simulink model "vco"  (R2019b)
settings: Solver=ode113  StartTime=0.0  StopTime=1e-6  RelTol=1e-3
values from neighbouring files (symbols this model uses):
  fs = fB*2    (= 10000000)    [vco_counter_m.m]    (also in vco_m.m = 1600000000)
  fvco = 1000e6    (= 1000000000)    [vco_counter_m.m]    (also in vco_m.m = 1600000000)
  ts = 1/fs    (= 1e-07)    [vco_counter_m.m]    (also in vco_m.m = 6.25e-10)
  tsys_res = 1e-11    [vco_counter_m.m]    (also in vco_m.m = 6.25e-10)
  tvco = 1/fvco    (= 6.25e-10)    [vco_m.m]
  vco_inverter_nums = 33    [vco_m.m]
libraries: simulink_extras x66
(part 2 of 2)

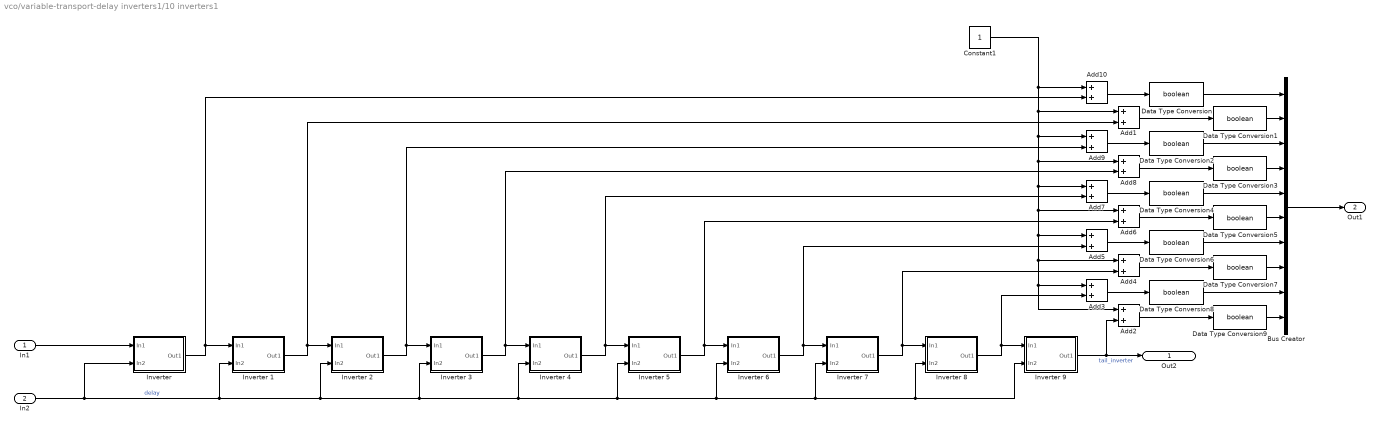
== system vco/variable-transport-delay inverters1/10 inverters1 ==
  In1 : Inport
  In2 : Inport  Port=2
  Add{1..10} (10 alike) : Sum
  Bus Creator : BusCreator  Inputs=10
  Constant1 : Constant  SampleTime=1e-11
  Data Type Conversion{,1..9} (10 alike) : DataTypeConversion  OutDataTypeStr=boolean
  "Inverter " : Subsystem
  Inverter 1 : Subsystem
  Inverter 2 : Subsystem
  Inverter 3 : Subsystem
  Inverter 4 : Subsystem
  Inverter 5 : Subsystem
  Inverter 6 : Subsystem
  Inverter 7 : Subsystem
  Inverter 8 : Subsystem
  Inverter 9 : Subsystem
  Out2 : Outport
  Out1 : Outport  Port=2
  wires:
  Bus Creator/1 -> Out1/1
  Add2/1 -> Data Type Conversion9/1
  Add3/1 -> Data Type Conversion8/1
  Add5/1 -> Data Type Conversion6/1
  Add4/1 -> Data Type Conversion7/1
  Add6/1 -> Data Type Conversion5/1
  Add9/1 -> Data Type Conversion2/1
  Add7/1 -> Data Type Conversion4/1
  Add8/1 -> Data Type Conversion3/1
  Add1/1 -> Data Type Conversion1/1
  Add10/1 -> Data Type Conversion/1
  Constant1/1 -> Add2/1, Add3/1, Add4/1, Add5/1, Add6/1, Add7/1, Add8/1, Add9/1, Add1/1, Add10/1
  Data Type Conversion/1 -> Bus Creator/1
  Data Type Conversion1/1 -> Bus Creator/2
  Data Type Conversion3/1 -> Bus Creator/4
  Data Type Conversion2/1 -> Bus Creator/3
  Data Type Conversion4/1 -> Bus Creator/5
  Data Type Conversion5/1 -> Bus Creator/6
  Data Type Conversion6/1 -> Bus Creator/7
  Data Type Conversion7/1 -> Bus Creator/8
  Data Type Conversion8/1 -> Bus Creator/9
  Data Type Conversion9/1 -> Bus Creator/10
  "Inverter "/1(Out1) -> Add10/2, Inverter 1/1(In1)
  Inverter 1/1(Out1) -> Add1/2, Inverter 2/1(In1)
  Inverter 2/1(Out1) -> Add9/2, Inverter 3/1(In1)
  Inverter 3/1(Out1) -> Add8/2, Inverter 4/1(In1)
  Inverter 4/1(Out1) -> Add7/2, Inverter 5/1(In1)
  Inverter 5/1(Out1) -> Add6/2, Inverter 6/1(In1)
  Inverter 6/1(Out1) -> Add5/2, Inverter 7/1(In1)
  Inverter 7/1(Out1) -> Add4/2, Inverter 8/1(In1)
  Inverter 8/1(Out1) -> Add3/2, Inverter 9/1(In1)
  In1/1 -> "Inverter "/1(In1)
  In2/1 -> Inverter 9/2(In2), Inverter 8/2(In2), Inverter 7/2(In2), Inverter 6/2(In2), Inverter 5/2(In2), Inverter 4/2(In2), Inverter 3/2(In2), Inverter 2/2(In2), Inverter 1/2(In2), "Inverter "/2(In2)  "delay"
  Inverter 9/1(Out1) -> Add2/2, Out2/1  "tail_inverter"

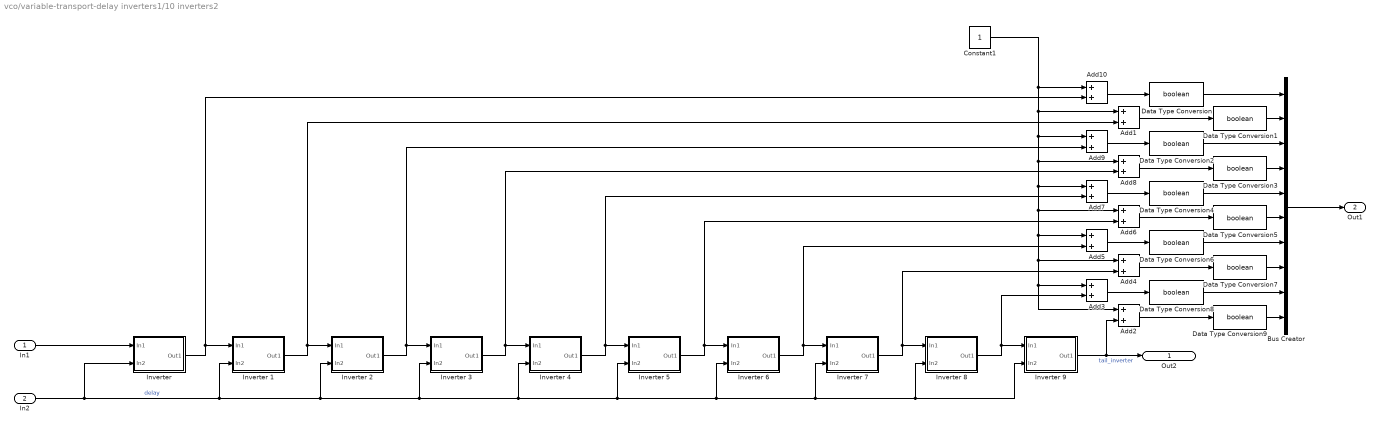
== system vco/variable-transport-delay inverters1/10 inverters2 ==
  In1 : Inport
  In2 : Inport  Port=2
  Add{1..10} (10 alike) : Sum
  Bus Creator : BusCreator  Inputs=10
  Constant1 : Constant  SampleTime=1e-11
  Data Type Conversion{,1..9} (10 alike) : DataTypeConversion  OutDataTypeStr=boolean
  "Inverter " : Subsystem
  Inverter 1 : Subsystem
  Inverter 2 : Subsystem
  Inverter 3 : Subsystem
  Inverter 4 : Subsystem
  Inverter 5 : Subsystem
  Inverter 6 : Subsystem
  Inverter 7 : Subsystem
  Inverter 8 : Subsystem
  Inverter 9 : Subsystem
  Out2 : Outport
  Out1 : Outport  Port=2
  wires:
  Bus Creator/1 -> Out1/1
  Add2/1 -> Data Type Conversion9/1
  Add3/1 -> Data Type Conversion8/1
  Add5/1 -> Data Type Conversion6/1
  Add4/1 -> Data Type Conversion7/1
  Add6/1 -> Data Type Conversion5/1
  Add9/1 -> Data Type Conversion2/1
  Add7/1 -> Data Type Conversion4/1
  Add8/1 -> Data Type Conversion3/1
  Add1/1 -> Data Type Conversion1/1
  Add10/1 -> Data Type Conversion/1
  Constant1/1 -> Add2/1, Add3/1, Add4/1, Add5/1, Add6/1, Add7/1, Add8/1, Add9/1, Add1/1, Add10/1
  Data Type Conversion/1 -> Bus Creator/1
  Data Type Conversion1/1 -> Bus Creator/2
  Data Type Conversion3/1 -> Bus Creator/4
  Data Type Conversion2/1 -> Bus Creator/3
  Data Type Conversion4/1 -> Bus Creator/5
  Data Type Conversion5/1 -> Bus Creator/6
  Data Type Conversion6/1 -> Bus Creator/7
  Data Type Conversion7/1 -> Bus Creator/8
  Data Type Conversion8/1 -> Bus Creator/9
  Data Type Conversion9/1 -> Bus Creator/10
  "Inverter "/1(Out1) -> Add10/2, Inverter 1/1(In1)
  Inverter 1/1(Out1) -> Add1/2, Inverter 2/1(In1)
  Inverter 2/1(Out1) -> Add9/2, Inverter 3/1(In1)
  Inverter 3/1(Out1) -> Add8/2, Inverter 4/1(In1)
  Inverter 4/1(Out1) -> Add7/2, Inverter 5/1(In1)
  Inverter 5/1(Out1) -> Add6/2, Inverter 6/1(In1)
  Inverter 6/1(Out1) -> Add5/2, Inverter 7/1(In1)
  Inverter 7/1(Out1) -> Add4/2, Inverter 8/1(In1)
  Inverter 8/1(Out1) -> Add3/2, Inverter 9/1(In1)
  In1/1 -> "Inverter "/1(In1)
  In2/1 -> Inverter 9/2(In2), Inverter 8/2(In2), Inverter 7/2(In2), Inverter 6/2(In2), Inverter 5/2(In2), Inverter 4/2(In2), Inverter 3/2(In2), Inverter 2/2(In2), Inverter 1/2(In2), "Inverter "/2(In2)  "delay"
  Inverter 9/1(Out1) -> Add2/2, Out2/1  "tail_inverter"

== system vco/variable-transport-delay inverters1/3 inverters ==
  In1 : Inport
  In2 : Inport  Port=2
  Add1 : Sum
  Add10 : Sum
  Add9 : Sum
  Bus Creator : BusCreator  Inputs=3
  Constant1 : Constant  SampleTime=1e-11
  Data Type Conversion : DataTypeConversion  OutDataTypeStr=boolean
  Data Type Conversion1 : DataTypeConversion  OutDataTypeStr=boolean
  Data Type Conversion2 : DataTypeConversion  OutDataTypeStr=boolean
  "Inverter " : Subsystem
  Inverter 1 : Subsystem
  Inverter 2 : Subsystem
  Out2 : Outport
  Out1 : Outport  Port=2
  wires:
  Bus Creator/1 -> Out1/1
  Add9/1 -> Data Type Conversion2/1
  Add1/1 -> Data Type Conversion1/1
  Add10/1 -> Data Type Conversion/1
  Constant1/1 -> Add9/1, Add1/1, Add10/1
  Data Type Conversion/1 -> Bus Creator/1
  Data Type Conversion1/1 -> Bus Creator/2
  Data Type Conversion2/1 -> Bus Creator/3
  "Inverter "/1(Out1) -> Add10/2, Inverter 1/1(In1)
  Inverter 1/1(Out1) -> Add1/2, Inverter 2/1(In1)
  Inverter 2/1(Out1) -> Out2/1, Add9/2  "tail_inverter"
  In1/1 -> "Inverter "/1(In1)
  In2/1 -> Inverter 2/2(In2), Inverter 1/2(In2), "Inverter "/2(In2)  "delay"

== system vco/variable-transport-delay inverters1/10 inverters/Inverter  ==
  In1 : Inport
  In2 : Inport  Port=2
  Constant3 : Constant  Value=-1  SampleTime=-1
  Constant4 : Constant  SampleTime=-1
  Integrator : Integrator  InitialCondition=1  LimitOutput=on  UpperSaturationLimit=1  LowerSaturationLimit=-1
  Product1 : Product
  Switch3 : Switch  Criteria=u2 > Threshold
  Out1 : Outport
  wires:
  Product1/1 -> Integrator/1
  Constant3/1 -> Switch3/1
  Constant4/1 -> Switch3/3
  Integrator/1 -> Switch3/2
  Switch3/1 -> Out1/1
  In1/1 -> Product1/1
  In2/1 -> Product1/2  "freq"

== system vco/variable-transport-delay inverters1/10 inverters/Inverter 1 ==
  In1 : Inport
  In2 : Inport  Port=2
  Constant3 : Constant  Value=-1  SampleTime=-1
  Constant4 : Constant  SampleTime=-1
  Integrator : Integrator  InitialCondition=-1  LimitOutput=on  UpperSaturationLimit=1  LowerSaturationLimit=-1
  Product1 : Product
  Switch3 : Switch  Criteria=u2 > Threshold
  Out1 : Outport
  wires:
  Product1/1 -> Integrator/1
  Constant3/1 -> Switch3/1
  Constant4/1 -> Switch3/3
  Integrator/1 -> Switch3/2
  Switch3/1 -> Out1/1
  In1/1 -> Product1/1
  In2/1 -> Product1/2  "freq"

== system vco/variable-transport-delay inverters1/10 inverters/Inverter 2 ==
  In1 : Inport
  In2 : Inport  Port=2
  Constant3 : Constant  Value=-1  SampleTime=-1
  Constant4 : Constant  SampleTime=-1
  Integrator : Integrator  InitialCondition=1  LimitOutput=on  UpperSaturationLimit=1  LowerSaturationLimit=-1
  Product1 : Product
  Switch3 : Switch  Criteria=u2 > Threshold
  Out1 : Outport
  wires:
  Product1/1 -> Integrator/1
  Constant3/1 -> Switch3/1
  Constant4/1 -> Switch3/3
  Integrator/1 -> Switch3/2
  Switch3/1 -> Out1/1
  In1/1 -> Product1/1
  In2/1 -> Product1/2  "freq"

== system vco/variable-transport-delay inverters1/10 inverters/Inverter 3 ==
  In1 : Inport
  In2 : Inport  Port=2
  Constant3 : Constant  Value=-1  SampleTime=-1
  Constant4 : Constant  SampleTime=-1
  Integrator : Integrator  InitialCondition=-1  LimitOutput=on  UpperSaturationLimit=1  LowerSaturationLimit=-1
  Product1 : Product
  Switch3 : Switch  Criteria=u2 > Threshold
  Out1 : Outport
  wires:
  Product1/1 -> Integrator/1
  Constant3/1 -> Switch3/1
  Constant4/1 -> Switch3/3
  Integrator/1 -> Switch3/2
  Switch3/1 -> Out1/1
  In1/1 -> Product1/1
  In2/1 -> Product1/2  "freq"

== system vco/variable-transport-delay inverters1/10 inverters/Inverter 4 ==
  In1 : Inport
  In2 : Inport  Port=2
  Constant3 : Constant  Value=-1  SampleTime=-1
  Constant4 : Constant  SampleTime=-1
  Integrator : Integrator  InitialCondition=1  LimitOutput=on  UpperSaturationLimit=1  LowerSaturationLimit=-1
  Product1 : Product
  Switch3 : Switch  Criteria=u2 > Threshold
  Out1 : Outport
  wires:
  Product1/1 -> Integrator/1
  Constant3/1 -> Switch3/1
  Constant4/1 -> Switch3/3
  Integrator/1 -> Switch3/2
  Switch3/1 -> Out1/1
  In1/1 -> Product1/1
  In2/1 -> Product1/2  "freq"

== system vco/variable-transport-delay inverters1/10 inverters/Inverter 5 ==
  In1 : Inport
  In2 : Inport  Port=2
  Constant3 : Constant  Value=-1  SampleTime=-1
  Constant4 : Constant  SampleTime=-1
  Integrator : Integrator  InitialCondition=-1  LimitOutput=on  UpperSaturationLimit=1  LowerSaturationLimit=-1
  Product1 : Product
  Switch3 : Switch  Criteria=u2 > Threshold
  Out1 : Outport
  wires:
  Product1/1 -> Integrator/1
  Constant3/1 -> Switch3/1
  Constant4/1 -> Switch3/3
  Integrator/1 -> Switch3/2
  Switch3/1 -> Out1/1
  In1/1 -> Product1/1
  In2/1 -> Product1/2  "freq"

== system vco/variable-transport-delay inverters1/10 inverters/Inverter 6 ==
  In1 : Inport
  In2 : Inport  Port=2
  Constant3 : Constant  Value=-1  SampleTime=-1
  Constant4 : Constant  SampleTime=-1
  Integrator : Integrator  InitialCondition=1  LimitOutput=on  UpperSaturationLimit=1  LowerSaturationLimit=-1
  Product1 : Product
  Switch3 : Switch  Criteria=u2 > Threshold
  Out1 : Outport
  wires:
  Product1/1 -> Integrator/1
  Constant3/1 -> Switch3/1
  Constant4/1 -> Switch3/3
  Integrator/1 -> Switch3/2
  Switch3/1 -> Out1/1
  In1/1 -> Product1/1
  In2/1 -> Product1/2  "freq"

== system vco/variable-transport-delay inverters1/10 inverters/Inverter 7 ==
  In1 : Inport
  In2 : Inport  Port=2
  Constant3 : Constant  Value=-1  SampleTime=-1
  Constant4 : Constant  SampleTime=-1
  Integrator : Integrator  InitialCondition=-1  LimitOutput=on  UpperSaturationLimit=1  LowerSaturationLimit=-1
  Product1 : Product
  Switch3 : Switch  Criteria=u2 > Threshold
  Out1 : Outport
  wires:
  Product1/1 -> Integrator/1
  Constant3/1 -> Switch3/1
  Constant4/1 -> Switch3/3
  Integrator/1 -> Switch3/2
  Switch3/1 -> Out1/1
  In1/1 -> Product1/1
  In2/1 -> Product1/2  "freq"

== system vco/variable-transport-delay inverters1/10 inverters/Inverter 8 ==
  In1 : Inport
  In2 : Inport  Port=2
  Constant3 : Constant  Value=-1  SampleTime=-1
  Constant4 : Constant  SampleTime=-1
  Integrator : Integrator  InitialCondition=1  LimitOutput=on  UpperSaturationLimit=1  LowerSaturationLimit=-1
  Product1 : Product
  Switch3 : Switch  Criteria=u2 > Threshold
  Out1 : Outport
  wires:
  Product1/1 -> Integrator/1
  Constant3/1 -> Switch3/1
  Constant4/1 -> Switch3/3
  Integrator/1 -> Switch3/2
  Switch3/1 -> Out1/1
  In1/1 -> Product1/1
  In2/1 -> Product1/2  "freq"

== system vco/variable-transport-delay inverters1/10 inverters/Inverter 9 ==
  In1 : Inport
  In2 : Inport  Port=2
  Constant3 : Constant  Value=-1  SampleTime=-1
  Constant4 : Constant  SampleTime=-1
  Integrator : Integrator  InitialCondition=-1  LimitOutput=on  UpperSaturationLimit=1  LowerSaturationLimit=-1
  Product1 : Product
  Switch3 : Switch  Criteria=u2 > Threshold
  Out1 : Outport
  wires:
  Product1/1 -> Integrator/1
  Constant3/1 -> Switch3/1
  Constant4/1 -> Switch3/3
  Integrator/1 -> Switch3/2
  Switch3/1 -> Out1/1
  In1/1 -> Product1/1
  In2/1 -> Product1/2  "freq"

== system vco/variable-transport-delay inverters1/10 inverters1/Inverter  ==
  In1 : Inport
  In2 : Inport  Port=2
  Constant3 : Constant  Value=-1  SampleTime=-1
  Constant4 : Constant  SampleTime=-1
  Integrator : Integrator  InitialCondition=1  LimitOutput=on  UpperSaturationLimit=1  LowerSaturationLimit=-1
  Product1 : Product
  Switch3 : Switch  Criteria=u2 > Threshold
  Out1 : Outport
  wires:
  Product1/1 -> Integrator/1
  Constant3/1 -> Switch3/1
  Constant4/1 -> Switch3/3
  Integrator/1 -> Switch3/2
  Switch3/1 -> Out1/1
  In1/1 -> Product1/1
  In2/1 -> Product1/2  "freq"

== system vco/variable-transport-delay inverters1/10 inverters1/Inverter 1 ==
  In1 : Inport
  In2 : Inport  Port=2
  Constant3 : Constant  Value=-1  SampleTime=-1
  Constant4 : Constant  SampleTime=-1
  Integrator : Integrator  InitialCondition=-1  LimitOutput=on  UpperSaturationLimit=1  LowerSaturationLimit=-1
  Product1 : Product
  Switch3 : Switch  Criteria=u2 > Threshold
  Out1 : Outport
  wires:
  Product1/1 -> Integrator/1
  Constant3/1 -> Switch3/1
  Constant4/1 -> Switch3/3
  Integrator/1 -> Switch3/2
  Switch3/1 -> Out1/1
  In1/1 -> Product1/1
  In2/1 -> Product1/2  "freq"

== system vco/variable-transport-delay inverters1/10 inverters1/Inverter 2 ==
  In1 : Inport
  In2 : Inport  Port=2
  Constant3 : Constant  Value=-1  SampleTime=-1
  Constant4 : Constant  SampleTime=-1
  Integrator : Integrator  InitialCondition=1  LimitOutput=on  UpperSaturationLimit=1  LowerSaturationLimit=-1
  Product1 : Product
  Switch3 : Switch  Criteria=u2 > Threshold
  Out1 : Outport
  wires:
  Product1/1 -> Integrator/1
  Constant3/1 -> Switch3/1
  Constant4/1 -> Switch3/3
  Integrator/1 -> Switch3/2
  Switch3/1 -> Out1/1
  In1/1 -> Product1/1
  In2/1 -> Product1/2  "freq"

== system vco/variable-transport-delay inverters1/10 inverters1/Inverter 3 ==
  In1 : Inport
  In2 : Inport  Port=2
  Constant3 : Constant  Value=-1  SampleTime=-1
  Constant4 : Constant  SampleTime=-1
  Integrator : Integrator  InitialCondition=-1  LimitOutput=on  UpperSaturationLimit=1  LowerSaturationLimit=-1
  Product1 : Product
  Switch3 : Switch  Criteria=u2 > Threshold
  Out1 : Outport
  wires:
  Product1/1 -> Integrator/1
  Constant3/1 -> Switch3/1
  Constant4/1 -> Switch3/3
  Integrator/1 -> Switch3/2
  Switch3/1 -> Out1/1
  In1/1 -> Product1/1
  In2/1 -> Product1/2  "freq"

== system vco/variable-transport-delay inverters1/10 inverters1/Inverter 4 ==
  In1 : Inport
  In2 : Inport  Port=2
  Constant3 : Constant  Value=-1  SampleTime=-1
  Constant4 : Constant  SampleTime=-1
  Integrator : Integrator  InitialCondition=1  LimitOutput=on  UpperSaturationLimit=1  LowerSaturationLimit=-1
  Product1 : Product
  Switch3 : Switch  Criteria=u2 > Threshold
  Out1 : Outport
  wires:
  Product1/1 -> Integrator/1
  Constant3/1 -> Switch3/1
  Constant4/1 -> Switch3/3
  Integrator/1 -> Switch3/2
  Switch3/1 -> Out1/1
  In1/1 -> Product1/1
  In2/1 -> Product1/2  "freq"

== system vco/variable-transport-delay inverters1/10 inverters1/Inverter 5 ==
  In1 : Inport
  In2 : Inport  Port=2
  Constant3 : Constant  Value=-1  SampleTime=-1
  Constant4 : Constant  SampleTime=-1
  Integrator : Integrator  InitialCondition=-1  LimitOutput=on  UpperSaturationLimit=1  LowerSaturationLimit=-1
  Product1 : Product
  Switch3 : Switch  Criteria=u2 > Threshold
  Out1 : Outport
  wires:
  Product1/1 -> Integrator/1
  Constant3/1 -> Switch3/1
  Constant4/1 -> Switch3/3
  Integrator/1 -> Switch3/2
  Switch3/1 -> Out1/1
  In1/1 -> Product1/1
  In2/1 -> Product1/2  "freq"

== system vco/variable-transport-delay inverters1/10 inverters1/Inverter 6 ==
  In1 : Inport
  In2 : Inport  Port=2
  Constant3 : Constant  Value=-1  SampleTime=-1
  Constant4 : Constant  SampleTime=-1
  Integrator : Integrator  InitialCondition=1  LimitOutput=on  UpperSaturationLimit=1  LowerSaturationLimit=-1
  Product1 : Product
  Switch3 : Switch  Criteria=u2 > Threshold
  Out1 : Outport
  wires:
  Product1/1 -> Integrator/1
  Constant3/1 -> Switch3/1
  Constant4/1 -> Switch3/3
  Integrator/1 -> Switch3/2
  Switch3/1 -> Out1/1
  In1/1 -> Product1/1
  In2/1 -> Product1/2  "freq"

== system vco/variable-transport-delay inverters1/10 inverters1/Inverter 7 ==
  In1 : Inport
  In2 : Inport  Port=2
  Constant3 : Constant  Value=-1  SampleTime=-1
  Constant4 : Constant  SampleTime=-1
  Integrator : Integrator  InitialCondition=-1  LimitOutput=on  UpperSaturationLimit=1  LowerSaturationLimit=-1
  Product1 : Product
  Switch3 : Switch  Criteria=u2 > Threshold
  Out1 : Outport
  wires:
  Product1/1 -> Integrator/1
  Constant3/1 -> Switch3/1
  Constant4/1 -> Switch3/3
  Integrator/1 -> Switch3/2
  Switch3/1 -> Out1/1
  In1/1 -> Product1/1
  In2/1 -> Product1/2  "freq"

== system vco/variable-transport-delay inverters1/10 inverters1/Inverter 8 ==
  In1 : Inport
  In2 : Inport  Port=2
  Constant3 : Constant  Value=-1  SampleTime=-1
  Constant4 : Constant  SampleTime=-1
  Integrator : Integrator  InitialCondition=1  LimitOutput=on  UpperSaturationLimit=1  LowerSaturationLimit=-1
  Product1 : Product
  Switch3 : Switch  Criteria=u2 > Threshold
  Out1 : Outport
  wires:
  Product1/1 -> Integrator/1
  Constant3/1 -> Switch3/1
  Constant4/1 -> Switch3/3
  Integrator/1 -> Switch3/2
  Switch3/1 -> Out1/1
  In1/1 -> Product1/1
  In2/1 -> Product1/2  "freq"

== system vco/variable-transport-delay inverters1/10 inverters1/Inverter 9 ==
  In1 : Inport
  In2 : Inport  Port=2
  Constant3 : Constant  Value=-1  SampleTime=-1
  Constant4 : Constant  SampleTime=-1
  Integrator : Integrator  InitialCondition=-1  LimitOutput=on  UpperSaturationLimit=1  LowerSaturationLimit=-1
  Product1 : Product
  Switch3 : Switch  Criteria=u2 > Threshold
  Out1 : Outport
  wires:
  Product1/1 -> Integrator/1
  Constant3/1 -> Switch3/1
  Constant4/1 -> Switch3/3
  Integrator/1 -> Switch3/2
  Switch3/1 -> Out1/1
  In1/1 -> Product1/1
  In2/1 -> Product1/2  "freq"

== system vco/variable-transport-delay inverters1/10 inverters2/Inverter  ==
  In1 : Inport
  In2 : Inport  Port=2
  Constant3 : Constant  Value=-1  SampleTime=-1
  Constant4 : Constant  SampleTime=-1
  Integrator : Integrator  InitialCondition=1  LimitOutput=on  UpperSaturationLimit=1  LowerSaturationLimit=-1
  Product1 : Product
  Switch3 : Switch  Criteria=u2 > Threshold
  Out1 : Outport
  wires:
  Product1/1 -> Integrator/1
  Constant3/1 -> Switch3/1
  Constant4/1 -> Switch3/3
  Integrator/1 -> Switch3/2
  Switch3/1 -> Out1/1
  In1/1 -> Product1/1
  In2/1 -> Product1/2  "freq"

== system vco/variable-transport-delay inverters1/10 inverters2/Inverter 1 ==
  In1 : Inport
  In2 : Inport  Port=2
  Constant3 : Constant  Value=-1  SampleTime=-1
  Constant4 : Constant  SampleTime=-1
  Integrator : Integrator  InitialCondition=-1  LimitOutput=on  UpperSaturationLimit=1  LowerSaturationLimit=-1
  Product1 : Product
  Switch3 : Switch  Criteria=u2 > Threshold
  Out1 : Outport
  wires:
  Product1/1 -> Integrator/1
  Constant3/1 -> Switch3/1
  Constant4/1 -> Switch3/3
  Integrator/1 -> Switch3/2
  Switch3/1 -> Out1/1
  In1/1 -> Product1/1
  In2/1 -> Product1/2  "freq"

== system vco/variable-transport-delay inverters1/10 inverters2/Inverter 2 ==
  In1 : Inport
  In2 : Inport  Port=2
  Constant3 : Constant  Value=-1  SampleTime=-1
  Constant4 : Constant  SampleTime=-1
  Integrator : Integrator  InitialCondition=1  LimitOutput=on  UpperSaturationLimit=1  LowerSaturationLimit=-1
  Product1 : Product
  Switch3 : Switch  Criteria=u2 > Threshold
  Out1 : Outport
  wires:
  Product1/1 -> Integrator/1
  Constant3/1 -> Switch3/1
  Constant4/1 -> Switch3/3
  Integrator/1 -> Switch3/2
  Switch3/1 -> Out1/1
  In1/1 -> Product1/1
  In2/1 -> Product1/2  "freq"

== system vco/variable-transport-delay inverters1/10 inverters2/Inverter 3 ==
  In1 : Inport
  In2 : Inport  Port=2
  Constant3 : Constant  Value=-1  SampleTime=-1
  Constant4 : Constant  SampleTime=-1
  Integrator : Integrator  InitialCondition=-1  LimitOutput=on  UpperSaturationLimit=1  LowerSaturationLimit=-1
  Product1 : Product
  Switch3 : Switch  Criteria=u2 > Threshold
  Out1 : Outport
  wires:
  Product1/1 -> Integrator/1
  Constant3/1 -> Switch3/1
  Constant4/1 -> Switch3/3
  Integrator/1 -> Switch3/2
  Switch3/1 -> Out1/1
  In1/1 -> Product1/1
  In2/1 -> Product1/2  "freq"

== system vco/variable-transport-delay inverters1/10 inverters2/Inverter 4 ==
  In1 : Inport
  In2 : Inport  Port=2
  Constant3 : Constant  Value=-1  SampleTime=-1
  Constant4 : Constant  SampleTime=-1
  Integrator : Integrator  InitialCondition=1  LimitOutput=on  UpperSaturationLimit=1  LowerSaturationLimit=-1
  Product1 : Product
  Switch3 : Switch  Criteria=u2 > Threshold
  Out1 : Outport
  wires:
  Product1/1 -> Integrator/1
  Constant3/1 -> Switch3/1
  Constant4/1 -> Switch3/3
  Integrator/1 -> Switch3/2
  Switch3/1 -> Out1/1
  In1/1 -> Product1/1
  In2/1 -> Product1/2  "freq"

== system vco/variable-transport-delay inverters1/10 inverters2/Inverter 5 ==
  In1 : Inport
  In2 : Inport  Port=2
  Constant3 : Constant  Value=-1  SampleTime=-1
  Constant4 : Constant  SampleTime=-1
  Integrator : Integrator  InitialCondition=-1  LimitOutput=on  UpperSaturationLimit=1  LowerSaturationLimit=-1
  Product1 : Product
  Switch3 : Switch  Criteria=u2 > Threshold
  Out1 : Outport
  wires:
  Product1/1 -> Integrator/1
  Constant3/1 -> Switch3/1
  Constant4/1 -> Switch3/3
  Integrator/1 -> Switch3/2
  Switch3/1 -> Out1/1
  In1/1 -> Product1/1
  In2/1 -> Product1/2  "freq"

== system vco/variable-transport-delay inverters1/10 inverters2/Inverter 6 ==
  In1 : Inport
  In2 : Inport  Port=2
  Constant3 : Constant  Value=-1  SampleTime=-1
  Constant4 : Constant  SampleTime=-1
  Integrator : Integrator  InitialCondition=1  LimitOutput=on  UpperSaturationLimit=1  LowerSaturationLimit=-1
  Product1 : Product
  Switch3 : Switch  Criteria=u2 > Threshold
  Out1 : Outport
  wires:
  Product1/1 -> Integrator/1
  Constant3/1 -> Switch3/1
  Constant4/1 -> Switch3/3
  Integrator/1 -> Switch3/2
  Switch3/1 -> Out1/1
  In1/1 -> Product1/1
  In2/1 -> Product1/2  "freq"

== system vco/variable-transport-delay inverters1/10 inverters2/Inverter 7 ==
  In1 : Inport
  In2 : Inport  Port=2
  Constant3 : Constant  Value=-1  SampleTime=-1
  Constant4 : Constant  SampleTime=-1
  Integrator : Integrator  InitialCondition=-1  LimitOutput=on  UpperSaturationLimit=1  LowerSaturationLimit=-1
  Product1 : Product
  Switch3 : Switch  Criteria=u2 > Threshold
  Out1 : Outport
  wires:
  Product1/1 -> Integrator/1
  Constant3/1 -> Switch3/1
  Constant4/1 -> Switch3/3
  Integrator/1 -> Switch3/2
  Switch3/1 -> Out1/1
  In1/1 -> Product1/1
  In2/1 -> Product1/2  "freq"

== system vco/variable-transport-delay inverters1/10 inverters2/Inverter 8 ==
  In1 : Inport
  In2 : Inport  Port=2
  Constant3 : Constant  Value=-1  SampleTime=-1
  Constant4 : Constant  SampleTime=-1
  Integrator : Integrator  InitialCondition=1  LimitOutput=on  UpperSaturationLimit=1  LowerSaturationLimit=-1
  Product1 : Product
  Switch3 : Switch  Criteria=u2 > Threshold
  Out1 : Outport
  wires:
  Product1/1 -> Integrator/1
  Constant3/1 -> Switch3/1
  Constant4/1 -> Switch3/3
  Integrator/1 -> Switch3/2
  Switch3/1 -> Out1/1
  In1/1 -> Product1/1
  In2/1 -> Product1/2  "freq"

== system vco/variable-transport-delay inverters1/10 inverters2/Inverter 9 ==
  In1 : Inport
  In2 : Inport  Port=2
  Constant3 : Constant  Value=-1  SampleTime=-1
  Constant4 : Constant  SampleTime=-1
  Integrator : Integrator  InitialCondition=-1  LimitOutput=on  UpperSaturationLimit=1  LowerSaturationLimit=-1
  Product1 : Product
  Switch3 : Switch  Criteria=u2 > Threshold
  Out1 : Outport
  wires:
  Product1/1 -> Integrator/1
  Constant3/1 -> Switch3/1
  Constant4/1 -> Switch3/3
  Integrator/1 -> Switch3/2
  Switch3/1 -> Out1/1
  In1/1 -> Product1/1
  In2/1 -> Product1/2  "freq"

== system vco/variable-transport-delay inverters1/3 inverters/Inverter  ==
  In1 : Inport
  In2 : Inport  Port=2
  Constant3 : Constant  Value=-1  SampleTime=-1
  Constant4 : Constant  SampleTime=-1
  Integrator : Integrator  InitialCondition=1  LimitOutput=on  UpperSaturationLimit=1  LowerSaturationLimit=-1
  Product1 : Product
  Switch3 : Switch  Criteria=u2 > Threshold
  Out1 : Outport
  wires:
  Product1/1 -> Integrator/1
  Constant3/1 -> Switch3/1
  Constant4/1 -> Switch3/3
  Integrator/1 -> Switch3/2
  Switch3/1 -> Out1/1
  In1/1 -> Product1/1
  In2/1 -> Product1/2  "freq"

== system vco/variable-transport-delay inverters1/3 inverters/Inverter 1 ==
  In1 : Inport
  In2 : Inport  Port=2
  Constant3 : Constant  Value=-1  SampleTime=-1
  Constant4 : Constant  SampleTime=-1
  Integrator : Integrator  InitialCondition=-1  LimitOutput=on  UpperSaturationLimit=1  LowerSaturationLimit=-1
  Product1 : Product
  Switch3 : Switch  Criteria=u2 > Threshold
  Out1 : Outport
  wires:
  Product1/1 -> Integrator/1
  Constant3/1 -> Switch3/1
  Constant4/1 -> Switch3/3
  Integrator/1 -> Switch3/2
  Switch3/1 -> Out1/1
  In1/1 -> Product1/1
  In2/1 -> Product1/2  "freq"

== system vco/variable-transport-delay inverters1/3 inverters/Inverter 2 ==
  In1 : Inport
  In2 : Inport  Port=2
  Constant3 : Constant  Value=-1  SampleTime=-1
  Constant4 : Constant  SampleTime=-1
  Integrator : Integrator  InitialCondition=1  LimitOutput=on  UpperSaturationLimit=1  LowerSaturationLimit=-1
  Product1 : Product
  Switch3 : Switch  Criteria=u2 > Threshold
  Out1 : Outport
  wires:
  Product1/1 -> Integrator/1
  Constant3/1 -> Switch3/1
  Constant4/1 -> Switch3/3
  Integrator/1 -> Switch3/2
  Switch3/1 -> Out1/1
  In1/1 -> Product1/1
  In2/1 -> Product1/2  "freq"
